simulink model "MMC_Control_PLECS_V2"  (R2018b)
settings: Solver=VariableStepAuto  StartTime=0.0  StopTime=0.1  FixedStep=sim_Ts  RelTol=1e-3
undefined symbols (not defined in the file): plecs
settings Model: Creator=jason  LastModifiedBy=jason

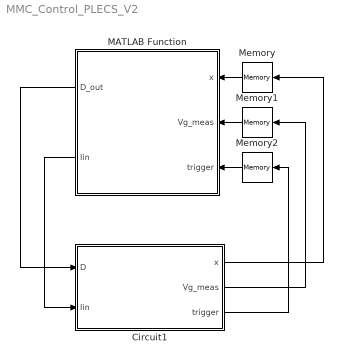
== system MMC_Control_PLECS_V2 ==
  Circuit1 : Subsystem  LoadFcn=plecs('sl', 200);  InitFcn=plecs('sl', 214);  StartFcn=plecs('sl', 208);  StopFcn=plecs('sl', 209);  mask(PlecsCircuit){PLECSData=<binary blob, 13548 chars, not shown>}
      mask prompts: PLECSData "PLECS Data (Do not delete or modify!)"
      mask init:
      | % PLACE CUSTOM INITIALIZATIONS ABOVE
      | % DO NOT REMOVE
      | plecs('sl', 215);
      | % DO NOT REMOVE
      settings: CopyFcn=plecs('sl', 203);  DeleteFcn=plecs('sl', 205);  UndoDeleteFcn=plecs('sl', 206);  PreSaveFcn=plecs('sl', 211);  PostSaveFcn=plecs('sl', 201);  NameChangeFcn=plecs('sl', 210);  DestroyFcn=plecs('sl', 207);  PreCopyFcn=plecs('sl', 216);  OpenFcn=plecs('sl', 202);  ErrorFcn=plerrorfcn
      mask Help: web(['file:///' fullfile(plecsdoc, 'creatingacircuit.html')])
      mask Display: disp('PLECS\nCircuit')
  MATLAB Function : MATLAB Function  TreatAsAtomicUnit=on
  Memory : Memory  InitialCondition=[50,50,50,4,4,4];  InheritSampleTime=on
  Memory1 : Memory  InitialCondition=[0,0,0];  InheritSampleTime=on
  Memory2 : Memory  InheritSampleTime=on
  wires:
  Circuit1/3(trigger) -> Memory2/1
  Circuit1/2(Vg_meas) -> Memory1/1
  Circuit1/1(x) -> Memory/1
  MATLAB Function/2(Iin) -> Circuit1/2(Iin)
  MATLAB Function/1(D_out) -> Circuit1/1(D)
  Memory/1 -> MATLAB Function/1(x)
  Memory1/1 -> MATLAB Function/2(Vg_meas)
  Memory2/1 -> MATLAB Function/3(trigger)

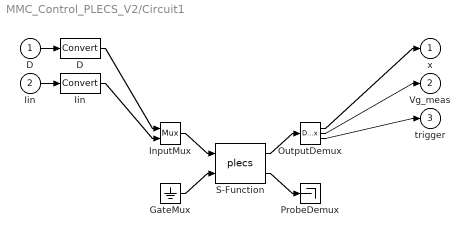
== system MMC_Control_PLECS_V2/Circuit1 ==
  D : Inport  PortDimensions=6
  Iin : Inport  Port=2  PortDimensions=3
  " D " : DataTypeConversion  SaturateOnIntegerOverflow=on  RndMeth=Zero
  " GateMux " : Ground
  " Iin " : DataTypeConversion  SaturateOnIntegerOverflow=on  RndMeth=Zero
  " InputMux " : Mux  Inputs=[ 6 3 ]
  " OutputDemux " : Demux  Outputs=[ 6 3 1 ]
  " ProbeDemux " : Terminator
  " S-Function " : S-Function  FunctionName=plecs  SFunctionDeploymentMode=off  EnableBusSupport=off
  x : Outport  PortDimensions=6
  Vg_meas : Outport  Port=2  PortDimensions=3
  trigger : Outport  Port=3  PortDimensions=1
  wires:
  " InputMux "/1 -> " S-Function "/1
  " GateMux "/1 -> " S-Function "/2
  " S-Function "/1 -> " OutputDemux "/1
  " S-Function "/2 -> " ProbeDemux "/1
  D/1 -> " D "/1
  " D "/1 -> " InputMux "/1
  Iin/1 -> " Iin "/1
  " Iin "/1 -> " InputMux "/2
  " OutputDemux "/1 -> x/1
  " OutputDemux "/2 -> Vg_meas/1
  " OutputDemux "/3 -> trigger/1

== matlab function MMC_Control_PLECS_V2/MATLAB Function ==
  data: x input; D_out output; Iin output; Vg_meas input; trigger input
function [D_out, Iin] = MMC_control(x, Vg_meas, trigger)

% % persistent err_int_var
% % if isempty(err_int_var)
% %     err_int_var = zeros(5,1);
% % end

persistent D_out_val err_int_val;
if isempty(D_out_val)
    D_out_val = [0.5; 0.5; 0.5; 0.5; 0.5; 0.5];
    err_int_val = zeros(5,1);
end

Ipv = 3;
Iin = [Ipv; Ipv; Ipv];

% Some nominal values 
Vpv  = 50; 
Ig = 4;
xnom = [Vpv,Vpv,Vpv,Ig,Ig,Ig]'; % six states to compensate


Ki = [946.470541106270,-78.9695483955200,84.3626063667173,-863.432464765911,1331.32266236245;133.979736482742,-129.901769191651,902.121155779121,-1509.12302944617,-694.645056439897;946.470541106269,84.3626063667193,-78.9695483955196,1331.32266236245,-863.432464765910;133.979736482743,902.121155779123,-129.901769191651,-694.645056439897,-1509.12302944617;-97.1036939308730,993.366963085425,124.676192876892,69.7914271799883,1450.06858130207;-97.1036939308747,124.676192876890,993.366963085427,1450.06858130207,69.7914271799855];
Kp = [-0.0454665586416772,-0.00199914482964152,0.00439942521823893,0.0718854631830432,-0.00534908518286846,-0.000795633659156228;0.00883038616267020,0.0110914315087384,-0.0332097516044704,0.0754302319385882,0.00331453961098084,0.00682158838613554;-0.0454665586416773,0.00439942521823883,-0.00199914482964147,-0.00534908518286850,0.0718854631830432,-0.000795633659156201;0.00883038616267014,-0.0332097516044704,0.0110914315087384,0.00331453961098087,0.0754302319385883,0.00682158838613551;-0.00208116300850227,-0.0492118673878262,0.00148788577326290,-0.000861248202244827,-0.00598010424054908,0.0633806439409333;-0.00208116300850226,0.00148788577326298,-0.0492118673878264,-0.00598010424054918,-0.000861248202244832,0.0633806439409334];

Igd = Vg_meas ./ 5.3333;
yd = [Vpv; Vpv; Vpv; Igd(1:2)]; % last point is not tracked (5 measurements to track)

tcy = 1/100e3;
D0 = [0.5; 0.5; 0.5; 0.5; 0.5; 0.5];

y = x(1:5);
state   =   x - xnom; 
err     =   yd - abs(y); % only care about absolute value 

err_int =   err*tcy  + err_int_val;
% simple anti-windup? 
err_int =  max(min(err_int,0.001),-0.001);


dD      = - Kp*state - Ki*err_int;
D       =   D0+dD;  % pay close attention to the sign!
% % D       =   max(min(D,0.999),0); % avoid saturation
D       =   max(min(D,0.9),0.1);
% % err_int_var = err_int_new;

if trigger
    D_out = D;
    D_out_val = D;
else
    D_out = D_out_val;
end

err_int_val = err_int;

end %function
